simulink model "MG1"  (R2023b)
settings: Solver=VariableStepAuto  StartTime=0.0  StopTime=100000.0  RelTol=1e-3
values from neighbouring files (symbols this model uses):
  n = 10    [Lab3_driver.m]
undefined symbols (not defined in the file or in its folder): m
settings Model: Creator=alberto  LastModifiedBy=alberto

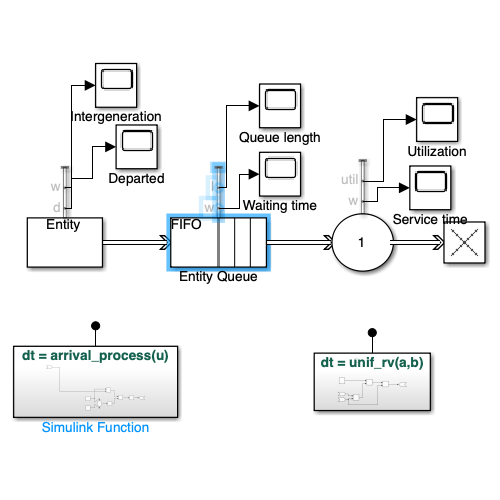
[thumbnail: Simulink's stored preview of the top-level diagram]
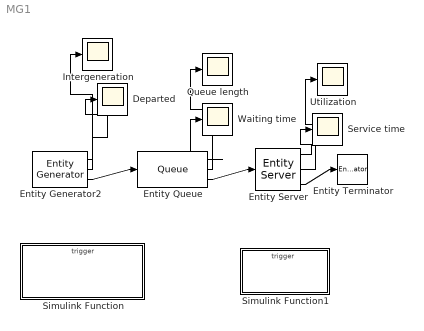
== system MG1 ==
  Departed : Scope
  Entity Generator2 : EntityGenerator  OutputPortMessageModes=n,n,m  TimeSource=MATLAB action  Period=0.5  IntergenerationTimeAction=dt = arrival_process(1/mG);  GenerateEntityAtSimulationStart=off  NumberEntitiesDeparted=on  AverageIntergenerationTime=on  EntityType=Structured  EntityTypeName=Entity
      settings: OutputPortMap=o0,o2,o3
  Entity Queue : Queue  InputPortMessageModes=m  OutputPortMessageModes=n,n,m  Capacity=Inf  AverageWait=on  AverageQueueLength=on
      settings: OutputPortMap=o2,o3,o5
  Entity Server : EntityServer  InputPortMessageModes=m  OutputPortMessageModes=n,n,m  Capacity=1  ServiceTimeSource=MATLAB action  ServiceTimeAction=dt = unif_rv(a,b);  AverageWait=on  Utilization=on
      settings: OutputPortMap=o4,o5,o9
  Entity Terminator : EntityTerminator  InputPortMessageModes=m
  Intergeneration : Scope
  Queue length : Scope
  Service time : Scope
  Simulink Function : Subsystem  TreatAsAtomicUnit=on
  Simulink Function1 : Subsystem  TreatAsAtomicUnit=on
  Utilization : Scope
  Waiting time : Scope
  wires:
  Entity Server/3 -> Entity Terminator/1
  Entity Queue/2 -> Queue length/1
  Entity Queue/3 -> Entity Server/1
  Entity Server/1 -> Service time/1
  Entity Generator2/2 -> Intergeneration/1
  Entity Generator2/1 -> Departed/1
  Entity Generator2/3 -> Entity Queue/1
  Entity Server/2 -> Utilization/1
  Entity Queue/1 -> Waiting time/1

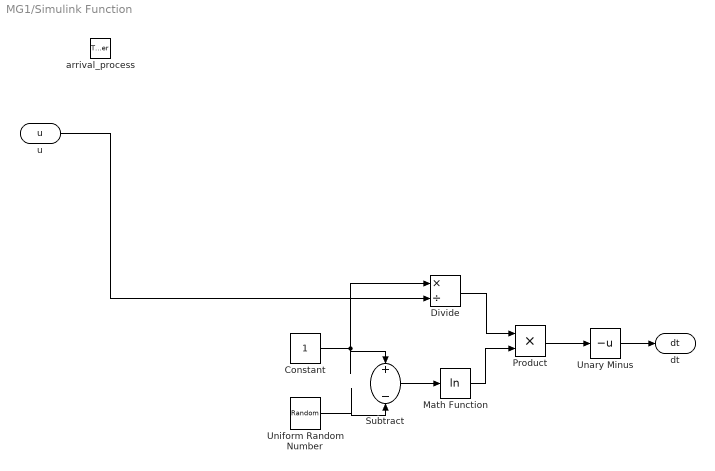
== system MG1/Simulink Function ==
  arrival_process : TriggerPort  TriggerType=function-call  IsSimulinkFunction=on  FunctionName=arrival_process  FunctionVisibility=scoped  VariantControl=(inherit)
  Constant : Constant
  Divide : Product  Inputs=*/
  Math Function : Math  Operator=log
  Product : Product
  Subtract : Sum  Inputs=+-
  Unary Minus : UnaryMinus
  Uniform Random Number : UniformRandomNumber  Minimum=0  Seed=randi(3333333)
  u : ArgIn  DisableCoverage=on  ArgumentName=u
  dt : ArgOut  DisableCoverage=on  ArgumentName=dt
  wires:
  Product/1 -> Unary Minus/1
  Constant/1 -> Divide/1, Subtract/1
  u/1 -> Divide/2
  Uniform Random Number/1 -> Subtract/2
  Divide/1 -> Product/1
  Math Function/1 -> Product/2
  Subtract/1 -> Math Function/1
  Unary Minus/1 -> dt/1

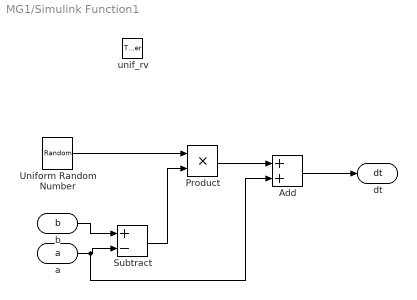
== system MG1/Simulink Function1 ==
  unif_rv : TriggerPort  TriggerType=function-call  IsSimulinkFunction=on  FunctionName=unif_rv  FunctionVisibility=scoped  VariantControl=(inherit)
  Add : Sum
  Product : Product
  Subtract : Sum  Inputs=+-
  Uniform Random Number : UniformRandomNumber  Minimum=0
  a : ArgIn  DisableCoverage=on  ArgumentName=a
  b : ArgIn  Port=2  ArgumentName=b
  dt : ArgOut  DisableCoverage=on  ArgumentName=dt
  wires:
  a/1 -> Add/2, Subtract/2
  b/1 -> Subtract/1
  Subtract/1 -> Product/2
  Uniform Random Number/1 -> Product/1
  Product/1 -> Add/1
  Add/1 -> dt/1
